simulink model "PI_sim"  (R2022b)
settings: Solver=VariableStepAuto  StartTime=0.0  StopTime=100  RelTol=1e-3
values from neighbouring files (symbols this model uses):
  k2a = k2(i)    [PI.m]    (also in kryt_jakosci.m)
settings Model: Creator=zuzanna  LastModifiedBy=zuzanna

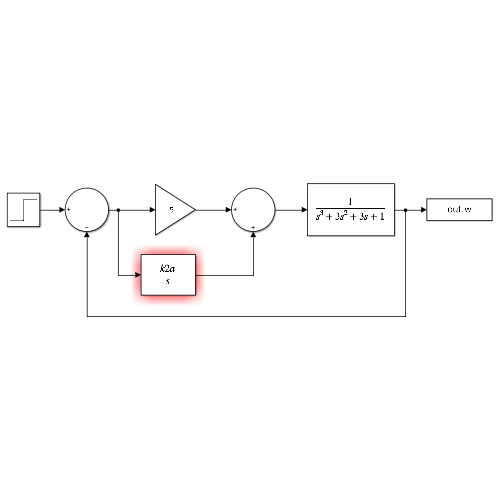
[thumbnail: Simulink's stored preview of the top-level diagram]
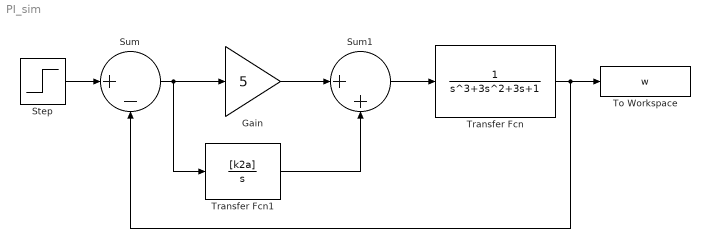
== system PI_sim ==
  Gain : Gain  Gain=5
  Step : Step  SampleTime=0
  Sum : Sum  Inputs=|+-
  Sum1 : Sum  Inputs=|++
  To Workspace : ToWorkspace  VariableName=w  SampleTime=-1
  Transfer Fcn : TransferFcn  Denominator=[1 3 3 1]
  Transfer Fcn1 : TransferFcn  Numerator=[k2a]  Denominator=[1 0]
  wires:
  Transfer Fcn/1 -> To Workspace/1, Sum/2
  Step/1 -> Sum/1
  Sum/1 -> Transfer Fcn1/1, Gain/1
  Transfer Fcn1/1 -> Sum1/2
  Gain/1 -> Sum1/1
  Sum1/1 -> Transfer Fcn/1
